simulink model "sim"  (R2016b)
settings: Solver=FixedStepDiscrete  StartTime=0  StopTime=Stoptime  FixedStep=0.1  RelTol=1e-3  EnableMultiTasking=on
values from neighbouring files (symbols this model uses):
  CYC_v = smooth(CYC_v,0.005 )    [main.m]
  ShiftDown = reshape(shift_down, [6,17])    [main.m]
  ShiftUp = reshape(shift_up, [5,17])    [main.m]
  VEH_M2 = 8700    [main.m]
undefined symbols (not defined in the file or in its folder): BrakeTorqueGain, CYC_gear, CYC_grade, CYC_t, DiscIntNeverNeededParam, DR_FF, DR_I, DR_P, Enable_Lag, Enable_Shift, ENG_Iei, Engine, Fr, g, ICE_maxT_T, ICE_maxT_w, Init, Powtrain_eff, sample_time, TC_Kfactor, TC_speedratio, TC_Torkratio, TRAN_gear, TRAN_ratio_diff, TRAN_ratio_gear, VEH_Cdl, VEH_M, VEH_Rw, WOT
libraries: simulink x2
settings Model: Creator=Dalaska  LastModifiedBy=daruiz
settings DataIOCC: LimitDataPoints=on  SaveFormat=Array
settings OptimizationCC: LifeSpan=inf
settings DebuggingCC: SFUnexpectedBacktrackingDiag=warning  SFNoUnconditionalDefaultTransitionDiag=warning  SFExecutionAtInitializationDiag=none
settings HardwareCC: ProdBitPerPointer=32  ProdBitPerSizeT=32  ProdBitPerPtrDiffT=32  ProdLargestAtomicFloat=None  ProdIntDivRoundTo=Undefined  ProdEndianess=Unspecified  ProdWordSize=32  ProdHWDeviceType=32-bit Generic
settings ModelReferenceCC: PropagateSignalLabelsOutOfModel=off
settings GRTTargetCC: TargetLangStandard=C89/C90 (ANSI)  GeneratePreprocessorConditionals=Disable all
settings ConfigComp: CovMetricSettings=dw  CovHtmlReporting=on  CovSaveCumulativeToWorkspaceVar=on  CovSaveSingleToWorkspaceVar=on  CovExternalEMLEnable=off

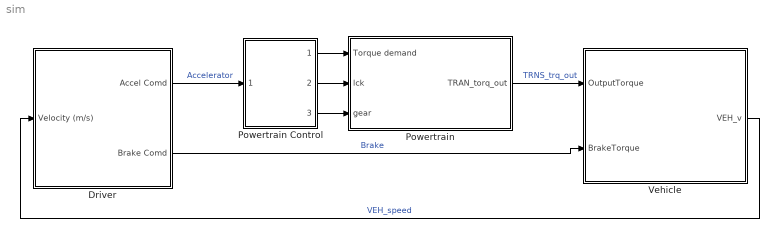
== system sim ==
  "Driver " : Subsystem
      mask Display: image(imread('Images\driver.jpg'))
  "Powertrain " : Subsystem
      mask Display: image(imread('Images\powertrain.jpg'))
  Powertrain Control : Subsystem
  Vehicle : Subsystem
      mask Display: image(imread('Images\truck.jpg'))
  wires:
  "Powertrain "/1(TRAN_torq_out) -> Vehicle/1(OutputTorque)  "TRNS_trq_out"
  "Driver "/1(Accel Comd) -> Powertrain Control/1(Throttle)  "Accelerator"
  Powertrain Control/1(ENG_torq) -> "Powertrain "/1(Torque demand)
  Powertrain Control/2(TC_lock) -> "Powertrain "/2(lck)
  Powertrain Control/3(TRAN_gear) -> "Powertrain "/3(gear)
  "Driver "/2(Brake Comd) -> Vehicle/2(BrakeTorque)  "Brake"
  Vehicle/1(VEH_v) -> "Driver "/1(Velocity (m/s))  "VEH_speed"

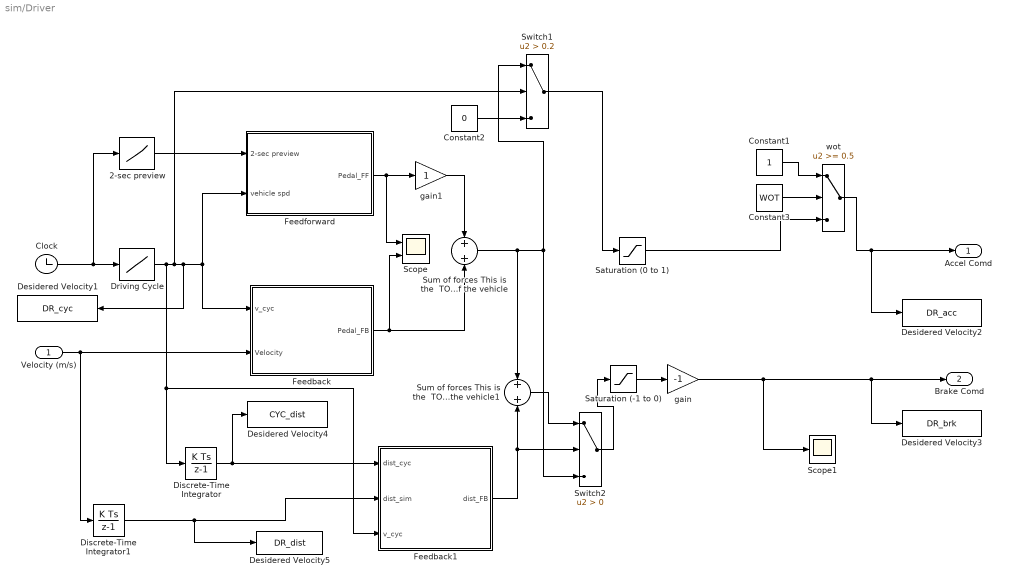
== system sim/Driver  ==
  Velocity (m/s) : Inport
  2-sec preview : Lookup  InputValues=CYC_t(1:length(CYC_t)-2)  Table=CYC_v(3:length(CYC_v))  SaturateOnIntegerOverflow=on
  Clock : Clock
  Constant1 : Constant
  Constant2 : Constant  Value=0
  Constant3 : Constant  Value=WOT
  Desidered Velocity1 : ToWorkspace  VariableName=DR_cyc  SaveFormat=Timeseries  SampleTime=-1
  Desidered Velocity2 : ToWorkspace  VariableName=DR_acc  SaveFormat=Timeseries  SampleTime=-1
  Desidered Velocity3 : ToWorkspace  VariableName=DR_brk  SaveFormat=Timeseries  SampleTime=-1
  Desidered Velocity4 : ToWorkspace  VariableName=CYC_dist  SaveFormat=Timeseries  SampleTime=-1
  Desidered Velocity5 : ToWorkspace  VariableName=DR_dist  SaveFormat=Timeseries  SampleTime=-1
  Discrete-Time Integrator : DiscreteIntegrator  InitialConditionSetting=State (most efficient)  SampleTime=sample_time  ICPrevOutput=DiscIntNeverNeededParam  ICPrevScaledInput=DiscIntNeverNeededParam
  Discrete-Time Integrator1 : DiscreteIntegrator  InitialConditionSetting=State (most efficient)  SampleTime=sample_time  ICPrevOutput=DiscIntNeverNeededParam  ICPrevScaledInput=DiscIntNeverNeededParam
  Driving Cycle : Lookup  InputValues=CYC_t  Table=CYC_v  SaturateOnIntegerOverflow=on
  Feedback : Subsystem
  Feedback1 : Subsystem
  Feedforward : Subsystem
  Saturation (-1 to 0) : Saturate  UpperLimit=0  LowerLimit=-1
  Saturation (0 to 1) : Saturate  UpperLimit=1  LowerLimit=0
  Scope : Scope  NumInputPorts=2
  Scope1 : Scope
  Sum of forces This is the  TOTAL force resisting forward motion of the vehicle : Sum  Tag=R12-1  SaturateOnIntegerOverflow=on  InputSameDT=on  OutDataTypeStr=Inherit: Same as first input
  Sum of forces This is the  TOTAL force resisting forward motion of the vehicle1 : Sum  Tag=R12-1  SaturateOnIntegerOverflow=on  InputSameDT=on  OutDataTypeStr=Inherit: Same as first input
  Switch1 : Switch  Criteria=u2 > Threshold  Threshold=0.2  SaturateOnIntegerOverflow=on  InputSameDT=on
  Switch2 : Switch  Criteria=u2 > Threshold  SaturateOnIntegerOverflow=on  InputSameDT=on
  gain : Gain  Gain=-1  SaturateOnIntegerOverflow=on  OutDataTypeStr=Inherit: Same as input  ParamDataTypeStr=Inherit: Same as input
  gain1 : Gain  SaturateOnIntegerOverflow=on  OutDataTypeStr=Inherit: Same as input  ParamDataTypeStr=Inherit: Same as input
  wot : Switch  Threshold=0.5
  Accel Comd : Outport  InitialOutput=0
  Brake Comd : Outport  Port=2  InitialOutput=0
  wires:
  Velocity (m/s)/1 -> Feedback/2(Velocity), Discrete-Time Integrator1/1
  Clock/1 -> 2-sec preview/1, Driving Cycle/1
  Driving Cycle/1 -> Switch1/2, Feedforward/2(vehicle spd), Feedback/1(v_cyc), Desidered Velocity1/1, Feedback1/3(v_cyc), Discrete-Time Integrator/1
  2-sec preview/1 -> Feedforward/1(2-sec preview)
  Feedforward/1(Pedal_FF) -> Scope/1, gain1/1
  Saturation (-1 to 0)/1 -> gain/1
  Feedback/1(Pedal_FB) -> Sum of forces This is the  TOTAL force resisting forward motion of the vehicle/2, Scope/2
  Discrete-Time Integrator/1 -> Desidered Velocity4/1, Feedback1/1(dist_cyc)
  Discrete-Time Integrator1/1 -> Feedback1/2(dist_sim), Desidered Velocity5/1
  Sum of forces This is the  TOTAL force resisting forward motion of the vehicle/1 -> Sum of forces This is the  TOTAL force resisting forward motion of the vehicle1/1, Switch1/1, Switch2/3
  gain/1 -> Scope1/1, Desidered Velocity3/1, Brake Comd/1
  gain1/1 -> Sum of forces This is the  TOTAL force resisting forward motion of the vehicle/1
  wot/1 -> Desidered Velocity2/1, Accel Comd/1
  Constant1/1 -> wot/1
  Constant3/1 -> wot/2
  Saturation (0 to 1)/1 -> wot/3
  Feedback1/1(dist_FB) -> Sum of forces This is the  TOTAL force resisting forward motion of the vehicle1/2, Switch2/2
  Sum of forces This is the  TOTAL force resisting forward motion of the vehicle1/1 -> Switch2/1
  Switch2/1 -> Saturation (-1 to 0)/1
  Switch1/1 -> Saturation (0 to 1)/1
  Constant2/1 -> Switch1/3

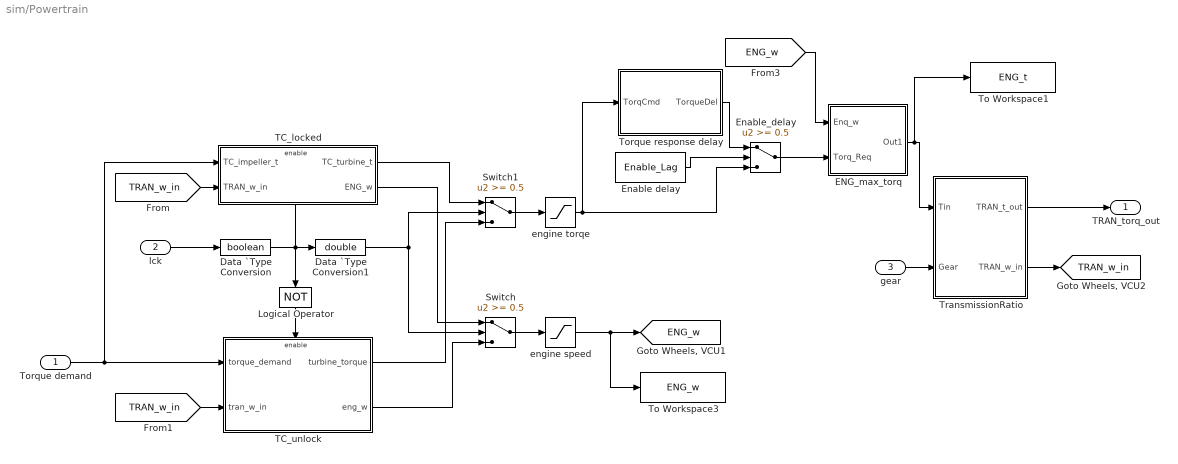
== system sim/Powertrain  ==
  Torque demand : Inport
  lck : Inport  Port=2
  gear : Inport  Port=3
  Data `Type Conversion : DataTypeConversion  OutDataTypeStr=boolean
  Data `Type Conversion1 : DataTypeConversion  OutDataTypeStr=double
  ENG_max_torq : Subsystem
  Enable delay : Constant  Value=Enable_Lag
  Enable_delay : Switch  Threshold=0.5
  Logical Operator : Logic  Operator=NOT  AllPortsSameDT=off  OutDataTypeStr=boolean
  Switch : Switch  Threshold=0.5
  Switch1 : Switch  Threshold=0.5
  TC_locked : Subsystem
  TC_unlock : Subsystem
  To Workspace1 : ToWorkspace  VariableName=ENG_t  SaveFormat=Timeseries  SampleTime=-1
  To Workspace3 : ToWorkspace  VariableName=ENG_w  SaveFormat=Timeseries  SampleTime=-1
  Torque response delay : Subsystem
  TransmissionRatio : Subsystem
  engine speed : Saturate  UpperLimit=2800  LowerLimit=700
  engine torqe : Saturate  UpperLimit=610  LowerLimit=0
  TRAN_torq_out : Outport
  tag scope: ENG_w=global, TRAN_w_in=global
  wires:
  gear/1 -> TransmissionRatio/2(Gear)
  TransmissionRatio/1("TRAN_t_out ") -> TRAN_torq_out/1
  lck/1 -> Data `Type Conversion/1
  TC_locked/2(ENG_w) -> Switch/1
  Data `Type Conversion/1 -> Logical Operator/1, Data `Type Conversion1/1, TC_locked/Enable
  Data `Type Conversion1/1 -> Switch/2, Switch1/2
  Logical Operator/1 -> TC_unlock/Enable
  TC_locked/1("TC_turbine_t ") -> Switch1/1
  TC_unlock/1(turbine_torque) -> Switch1/3
  TC_unlock/2(eng_w) -> Switch/3
  Switch/1 -> engine speed/1
  engine speed/1 -> [ENG_w], To Workspace3/1
  Torque demand/1 -> TC_locked/1(TC_impeller_t), TC_unlock/1(torque_demand)
  TransmissionRatio/2(TRAN_w_in) -> [TRAN_w_in]
  [TRAN_w_in] -> TC_locked/2(TRAN_w_in)
  [TRAN_w_in] -> TC_unlock/2(tran_w_in)
  ENG_max_torq/1(Out1) -> TransmissionRatio/1(Tin), To Workspace1/1
  Torque response delay/1(TorqueDel) -> Enable_delay/1
  Enable delay/1 -> Enable_delay/2
  [ENG_w] -> ENG_max_torq/1(Enq_w)
  Switch1/1 -> engine torqe/1
  Enable_delay/1 -> ENG_max_torq/2(Torq_Req)
  engine torqe/1 -> Enable_delay/3, Torque response delay/1(TorqCmd)

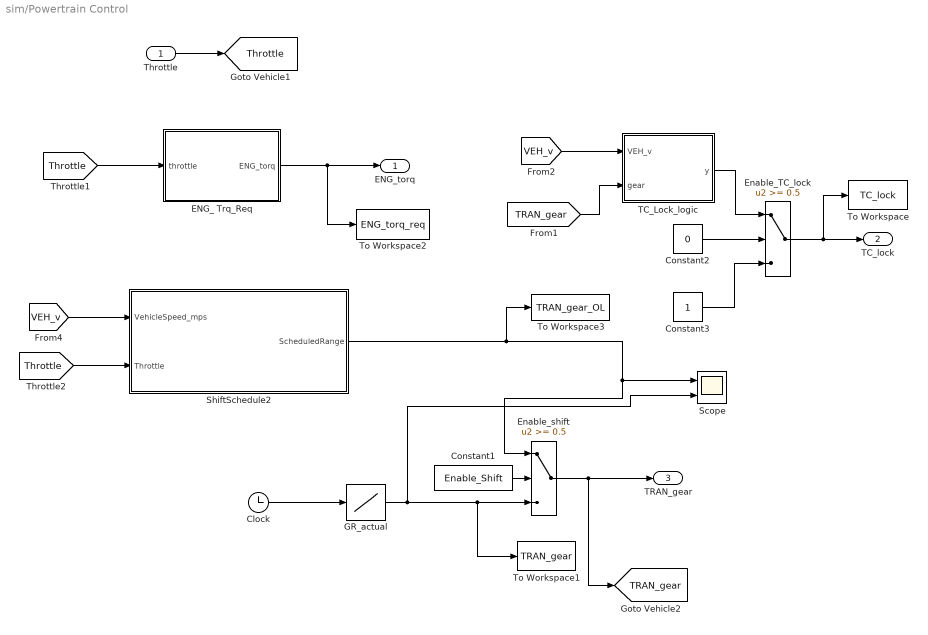
== system sim/Powertrain Control ==
  Throttle : Inport
  Clock : Clock
  Constant1 : Constant  Value=Enable_Shift
  Constant2 : Constant  Value=0
  Constant3 : Constant
  ENG_ Trq_Req : Subsystem
  Enable_TC_lock : Switch  Threshold=0.5
  Enable_shift : Switch  Threshold=0.5
  GR_actual : Lookup  InputValues=CYC_t  Table=CYC_gear  LookUpMeth=Use Input Nearest  SaturateOnIntegerOverflow=on
  Scope : Scope  NumInputPorts=2
  ShiftSchedule2 : Subsystem  TreatAsAtomicUnit=on
  TC_Lock_logic : MATLAB Function  TreatAsAtomicUnit=on
  To Workspace : ToWorkspace  VariableName=TC_lock  SaveFormat=Timeseries  SampleTime=-1
  To Workspace1 : ToWorkspace  VariableName=TRAN_gear  SaveFormat=Timeseries  SampleTime=-1
  To Workspace2 : ToWorkspace  VariableName=ENG_torq_req  SaveFormat=Timeseries  SampleTime=-1
  To Workspace3 : ToWorkspace  VariableName=TRAN_gear_OL  SaveFormat=Timeseries  SampleTime=-1
  ENG_torq : Outport
  TC_lock : Outport  Port=2
  TRAN_gear : Outport  Port=3
  tag scope: TRAN_gear=global, Throttle=global
  wires:
  Throttle/1 -> [Throttle]
  ENG_ Trq_Req/1(ENG_torq) -> ENG_torq/1, To Workspace2/1
  [VEH_v] -> TC_Lock_logic/1(VEH_v)
  Enable_shift/1 -> [TRAN_gear], TRAN_gear/1
  Clock/1 -> GR_actual/1
  GR_actual/1 -> Enable_shift/3, To Workspace1/1, Scope/2
  ShiftSchedule2/1(ScheduledRange) -> To Workspace3/1, Scope/1, Enable_shift/1
  Constant1/1 -> Enable_shift/2
  [TRAN_gear] -> TC_Lock_logic/2(gear)
  Constant3/1 -> Enable_TC_lock/3
  Enable_TC_lock/1 -> TC_lock/1, To Workspace/1
  Constant2/1 -> Enable_TC_lock/2
  TC_Lock_logic/1(y) -> Enable_TC_lock/1
  [Throttle] -> ENG_ Trq_Req/1(throttle)
  [VEH_v] -> ShiftSchedule2/1(VehicleSpeed_mps)
  [Throttle] -> ShiftSchedule2/2(Throttle)

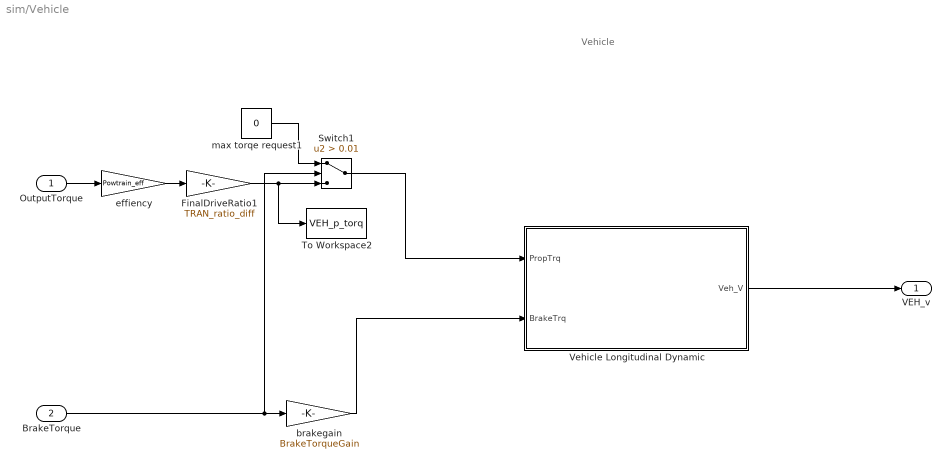
== system sim/Vehicle ==
  note: Vehicle
  OutputTorque : Inport
  BrakeTorque : Inport  Port=2
  FinalDriveRatio1 : Gain  Gain=TRAN_ratio_diff  SaturateOnIntegerOverflow=on  OutDataTypeStr=Inherit: Same as input  ParamDataTypeStr=Inherit: Same as input
  Switch1 : Switch  Criteria=u2 > Threshold  Threshold=0.01  ZeroCross=off
  To Workspace2 : ToWorkspace  VariableName=VEH_p_torq  SaveFormat=Timeseries  SampleTime=-1
  Vehicle Longitudinal Dynamic : Subsystem
  brakegain : Gain  Gain=BrakeTorqueGain  SaturateOnIntegerOverflow=on  OutDataTypeStr=Inherit: Same as input  ParamDataTypeStr=Inherit: Same as input
  effiency : Gain  Gain=Powtrain_eff  SaturateOnIntegerOverflow=on  OutDataTypeStr=Inherit: Same as input  ParamDataTypeStr=Inherit: Same as input
  max torqe request1 : Constant  Value=0  SampleTime=0
  VEH_v : Outport
  wires:
  OutputTorque/1 -> effiency/1
  BrakeTorque/1 -> Switch1/2, brakegain/1
  FinalDriveRatio1/1 -> To Workspace2/1, Switch1/3
  max torqe request1/1 -> Switch1/1
  effiency/1 -> FinalDriveRatio1/1
  Switch1/1 -> Vehicle Longitudinal Dynamic/1(PropTrq)
  brakegain/1 -> Vehicle Longitudinal Dynamic/2(BrakeTrq)
  Vehicle Longitudinal Dynamic/1(Veh_V) -> VEH_v/1

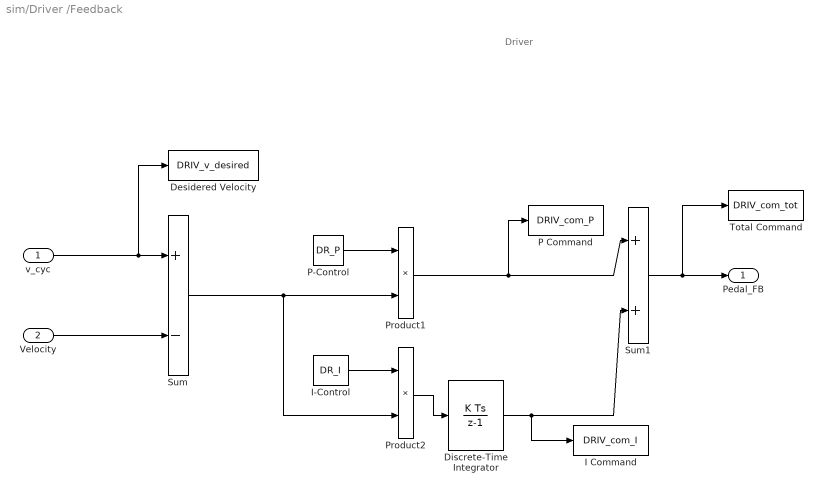
== system sim/Driver /Feedback ==
  note: Driver
  v_cyc : Inport
  Velocity : Inport  Port=2
  Desidered Velocity : ToWorkspace  VariableName=DRIV_v_desired  SampleTime=-1
  Discrete-Time Integrator : DiscreteIntegrator  InitialConditionSetting=State (most efficient)  SampleTime=sample_time  ICPrevOutput=DiscIntNeverNeededParam  ICPrevScaledInput=DiscIntNeverNeededParam
  I Command : ToWorkspace  VariableName=DRIV_com_I  SampleTime=-1
  I-Control : Constant  Value=DR_I
  P Command : ToWorkspace  VariableName=DRIV_com_P  SampleTime=-1
  P-Control : Constant  Value=DR_P
  Product1 : Product  RndMeth=Zero
  Product2 : Product  RndMeth=Zero
  Sum : Sum  Inputs=+-  SaturateOnIntegerOverflow=on  InputSameDT=on  OutDataTypeStr=Inherit: Same as first input
  Sum1 : Sum  SaturateOnIntegerOverflow=on  InputSameDT=on  OutDataTypeStr=Inherit: Same as first input
  Total Command : ToWorkspace  VariableName=DRIV_com_tot  SampleTime=-1
  Pedal_FB : Outport
  wires:
  Sum1/1 -> Total Command/1, Pedal_FB/1
  Sum/1 -> Product1/2, Product2/2
  Product1/1 -> Sum1/1, P Command/1
  Product2/1 -> Discrete-Time Integrator/1
  Discrete-Time Integrator/1 -> I Command/1, Sum1/2
  P-Control/1 -> Product1/1
  v_cyc/1 -> Sum/1, Desidered Velocity/1
  I-Control/1 -> Product2/1
  Velocity/1 -> Sum/2

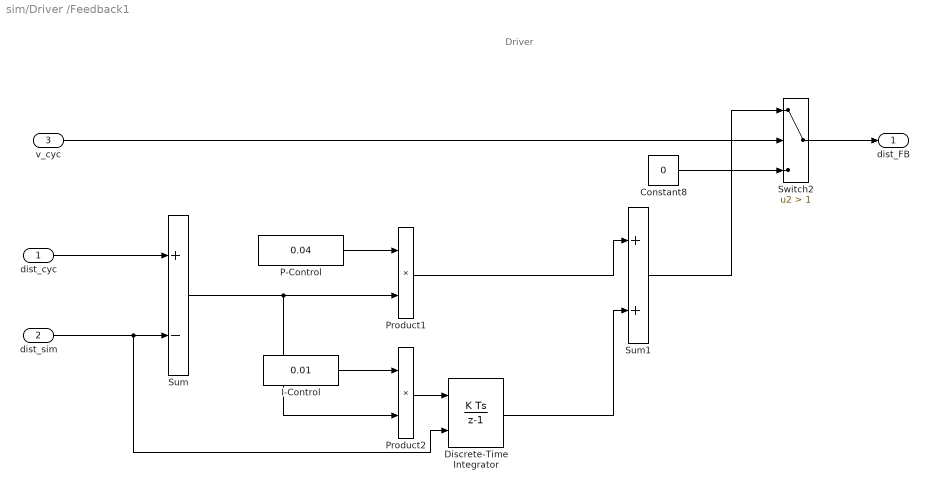
== system sim/Driver /Feedback1 ==
  note: Driver
  dist_cyc : Inport
  dist_sim : Inport  Port=2
  v_cyc : Inport  Port=3
  Constant8 : Constant  Value=0
  Discrete-Time Integrator : DiscreteIntegrator  ExternalReset=level  InitialConditionSetting=State (most efficient)  SampleTime=sample_time  ICPrevOutput=DiscIntNeverNeededParam  ICPrevScaledInput=DiscIntNeverNeededParam
  I-Control : Constant  Value=0.01
  P-Control : Constant  Value=0.04
  Product1 : Product  RndMeth=Zero
  Product2 : Product  RndMeth=Zero
  Sum : Sum  Inputs=+-  SaturateOnIntegerOverflow=on  InputSameDT=on  OutDataTypeStr=Inherit: Same as first input
  Sum1 : Sum  SaturateOnIntegerOverflow=on  InputSameDT=on  OutDataTypeStr=Inherit: Same as first input
  Switch2 : Switch  Criteria=u2 > Threshold  Threshold=1  SaturateOnIntegerOverflow=on  InputSameDT=on
  dist_FB : Outport
  wires:
  dist_sim/1 -> Discrete-Time Integrator/2, Sum/2
  Sum/1 -> Product1/2, Product2/2
  Product1/1 -> Sum1/1
  Product2/1 -> Discrete-Time Integrator/1
  Discrete-Time Integrator/1 -> Sum1/2
  P-Control/1 -> Product1/1
  dist_cyc/1 -> Sum/1
  I-Control/1 -> Product2/1
  v_cyc/1 -> Switch2/2
  Switch2/1 -> dist_FB/1
  Constant8/1 -> Switch2/3
  Sum1/1 -> Switch2/1

== system sim/Driver /Feedforward ==
  2-sec preview : Inport
  vehicle spd : Inport  Port=2
  Preview Gain : Gain  Gain=DR_FF  SaturateOnIntegerOverflow=on  OutDataTypeStr=Inherit: Same as input  ParamDataTypeStr=Inherit: Same as input
  Sum1 : Sum  Inputs=|+-  SaturateOnIntegerOverflow=on  InputSameDT=on  OutDataTypeStr=Inherit: Same as first input
  Pedal_FF : Outport
  wires:
  2-sec preview/1 -> Sum1/1
  Sum1/1 -> Preview Gain/1
  Preview Gain/1 -> Pedal_FF/1
  vehicle spd/1 -> Sum1/2

== system sim/Powertrain /ENG_max_torq ==
  Enq_w : Inport
  Torq_Req : Inport  Port=2
  Constant3 : Constant  Value=0
  ICE Max Torque Curve : Lookup  InputValues=ICE_maxT_w  Table=ICE_maxT_T  SaturateOnIntegerOverflow=on
  Saturation Dynamic : simulink/Discontinuities/Saturation Dynamic  OutMin=[]  OutMax=[]  OutDataTypeStr=Inherit: Same as second input  OutDataType=sfix(16)  OutScaling=2^-10  DoSatur=off
  rpm 2 rad/sec : Gain  Gain=pi*2/60
  Out1 : Outport
  wires:
  Saturation Dynamic/1 -> Out1/1
  rpm 2 rad/sec/1 -> ICE Max Torque Curve/1
  Constant3/1 -> Saturation Dynamic/3
  ICE Max Torque Curve/1 -> Saturation Dynamic/1
  Torq_Req/1 -> Saturation Dynamic/2
  Enq_w/1 -> rpm 2 rad/sec/1

== system sim/Powertrain /TC_locked ==
  TC_impeller_t : Inport
  TRAN_w_in : Inport  Port=2
  Enable : EnablePort  StatesWhenEnabling=reset  PropagateVarSize=During execution
  "TC_turbine_t " : Outport
  ENG_w : Outport  Port=2
  wires:
  TC_impeller_t/1 -> "TC_turbine_t "/1
  TRAN_w_in/1 -> ENG_w/1

== system sim/Powertrain /TC_unlock ==
  torque_demand : Inport
  tran_w_in : Inport  Port=2
  Enable : EnablePort  StatesWhenEnabling=reset  PropagateVarSize=During execution
  TC : Subsystem
  engine : Subsystem
  turbine_torque : Outport
  eng_w : Outport  Port=2
  wires:
  torque_demand/1 -> engine/2(Torque_Demand)
  TC/1("TC_impeller_t ") -> engine/1(Torque_Break)
  engine/1(ENG_w) -> eng_w/1, TC/1(TC_impeller_w)
  TC/2("TC_turbine_t ") -> turbine_torque/1  "TurbineTorque"
  tran_w_in/1 -> TC/2(TC_trub_w)

== system sim/Powertrain /Torque response delay ==
  TorqCmd : Inport  OutDataTypeStr=double  PortDimensions=1
  1-D Lookup Table : Lookup_n-D  NumberOfTableDimensions=1  BreakpointsForDimension1=[600 1200]  Table=[.8333 .8333]  ExtrapMethod=Clip  UseLastTableValue=on  RndMeth=Simplest  InputSameDT=on
  1-D Lookup Table1 : Lookup_n-D  NumberOfTableDimensions=1  BreakpointsForDimension1=[-.1 500]  Table=[10 .8333]  ExtrapMethod=Clip  UseLastTableValue=on  RndMeth=Simplest  InputSameDT=on
  Constant : Constant  Value=10  OutDataTypeStr=double
  Discrete Transfer Fcn (need to update coefficients) : DiscreteTransferFcn  Numerator=Engine.TorqResponseFltrNum  Denominator=Engine.TorqResponseFltrDen  SampleTime=sample_time
  Relational Operator : RelationalOperator  Operator=<=  OutDataTypeStr=boolean  RndMeth=Nearest
  Select Max : MinMax  Function=max  Inputs=2
  Switch : Switch  Criteria=u2 ~= 0
  Variable Rate Discrete Lag Filter : Subsystem
  TorqueDel : Outport
  wires:
  Variable Rate Discrete Lag Filter/1(Output) -> TorqueDel/1, 1-D Lookup Table1/1, Discrete Transfer Fcn (need to update coefficients)/1
  TorqCmd/1 -> Relational Operator/1, Variable Rate Discrete Lag Filter/1(Input)
  Discrete Transfer Fcn (need to update coefficients)/1 -> 1-D Lookup Table/1, Relational Operator/2
  Switch/1 -> Variable Rate Discrete Lag Filter/2(wn)
  Relational Operator/1 -> Switch/2
  Constant/1 -> Switch/1
  1-D Lookup Table/1 -> Select Max/2
  Select Max/1 -> Switch/3
  1-D Lookup Table1/1 -> Select Max/1

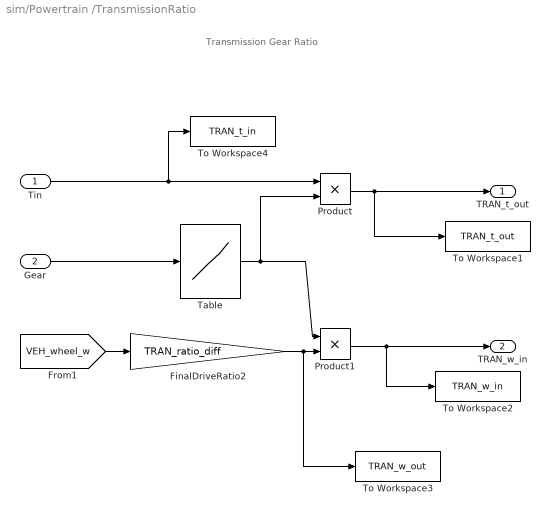
== system sim/Powertrain /TransmissionRatio ==
  note: Transmission Gear Ratio
  Tin : Inport
  Gear : Inport  Port=2
  FinalDriveRatio2 : Gain  Gain=TRAN_ratio_diff  SaturateOnIntegerOverflow=on  OutDataTypeStr=Inherit: Same as input  ParamDataTypeStr=Inherit: Same as input
  Product : Product  SaturateOnIntegerOverflow=on  InputSameDT=on  OutDataTypeStr=Inherit: Same as first input
  Product1 : Product  SaturateOnIntegerOverflow=on  InputSameDT=on  OutDataTypeStr=Inherit: Same as first input
  Table : Lookup_n-D  NumberOfTableDimensions=1  BreakpointsForDimension1=TRAN_gear  Table=TRAN_ratio_gear  OutDataTypeStr=double  SaturateOnIntegerOverflow=on  InputSameDT=on  LockScale=on
  To Workspace1 : ToWorkspace  VariableName=TRAN_t_out  SaveFormat=Timeseries  SampleTime=-1
  To Workspace2 : ToWorkspace  VariableName=TRAN_w_in  SaveFormat=Timeseries  SampleTime=-1
  To Workspace3 : ToWorkspace  VariableName=TRAN_w_out  SaveFormat=Timeseries  SampleTime=-1
  To Workspace4 : ToWorkspace  VariableName=TRAN_t_in  SaveFormat=Timeseries  SampleTime=-1
  "TRAN_t_out " : Outport
  TRAN_w_in : Outport  Port=2
  wires:
  Table/1 -> Product1/1, Product/2
  Tin/1 -> To Workspace4/1, Product/1
  Gear/1 -> Table/1
  [VEH_wheel_w] -> FinalDriveRatio2/1
  Product/1 -> To Workspace1/1, "TRAN_t_out "/1
  FinalDriveRatio2/1 -> To Workspace3/1, Product1/2
  Product1/1 -> TRAN_w_in/1, To Workspace2/1

== system sim/Powertrain Control/ENG_ Trq_Req ==
  throttle : Inport
  ENG_max_torq : Subsystem
  Max_torqe_request : Constant  Value=620
  Memory : Memory
  Product3 : Product  RndMeth=Zero
  ENG_torq : Outport
  wires:
  [ENG_w] -> Memory/1
  Memory/1 -> ENG_max_torq/1(Enq_w)
  throttle/1 -> Product3/1
  ENG_max_torq/1(Out1) -> ENG_torq/1
  Max_torqe_request/1 -> Product3/2
  Product3/1 -> ENG_max_torq/2(Torq_Req)

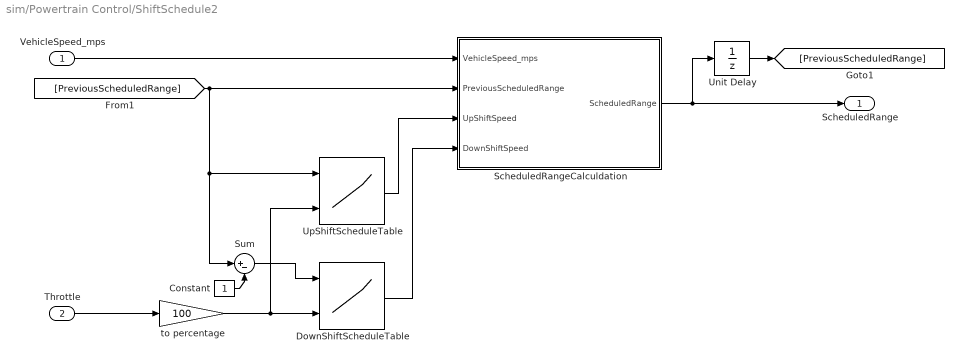
== system sim/Powertrain Control/ShiftSchedule2 ==
  VehicleSpeed_mps : Inport  OutDataTypeStr=double  PortDimensions=1
  Throttle : Inport  Port=2  OutDataTypeStr=double  PortDimensions=1
  Constant : Constant
  DownShiftScheduleTable : Lookup_n-D  BreakpointsForDimension1=[0:1:5]  BreakpointsForDimension2=[0:6.25:100]  BeginIndexSearchUsingPreviousIndexResult=on  Table=ShiftDown  ExtrapMethod=Clip  UseLastTableValue=on  RndMeth=Simplest  InputSameDT=on
  ScheduledRangeCalculdation : Subsystem  TreatAsAtomicUnit=on
  Sum : Sum  Inputs=|+-
  Unit Delay : UnitDelay  InitialCondition=1  SampleTime=-1
  UpShiftScheduleTable : Lookup_n-D  BreakpointsForDimension1=[1:1:5]  BreakpointsForDimension2=[0:6.25:100]  BeginIndexSearchUsingPreviousIndexResult=on  Table=ShiftUp  ExtrapMethod=Clip  UseLastTableValue=on  RndMeth=Simplest  InputSameDT=on
  to percentage : Gain  Gain=100  SaturateOnIntegerOverflow=on  OutDataTypeStr=Inherit: Same as input  ParamDataTypeStr=Inherit: Same as input
  ScheduledRange : Outport  OutDataTypeStr=double  PortDimensions=1
  wires:
  ScheduledRangeCalculdation/1(ScheduledRange) -> Unit Delay/1, ScheduledRange/1
  VehicleSpeed_mps/1 -> ScheduledRangeCalculdation/1(VehicleSpeed_mps)
  DownShiftScheduleTable/1 -> ScheduledRangeCalculdation/4(DownShiftSpeed)
  UpShiftScheduleTable/1 -> ScheduledRangeCalculdation/3(UpShiftSpeed)
  Throttle/1 -> to percentage/1
  to percentage/1 -> UpShiftScheduleTable/2, DownShiftScheduleTable/2
  Unit Delay/1 -> [PreviousScheduledRange]
  [PreviousScheduledRange] -> ScheduledRangeCalculdation/2(PreviousScheduledRange), Sum/1, UpShiftScheduleTable/1
  Sum/1 -> DownShiftScheduleTable/1
  Constant/1 -> Sum/2

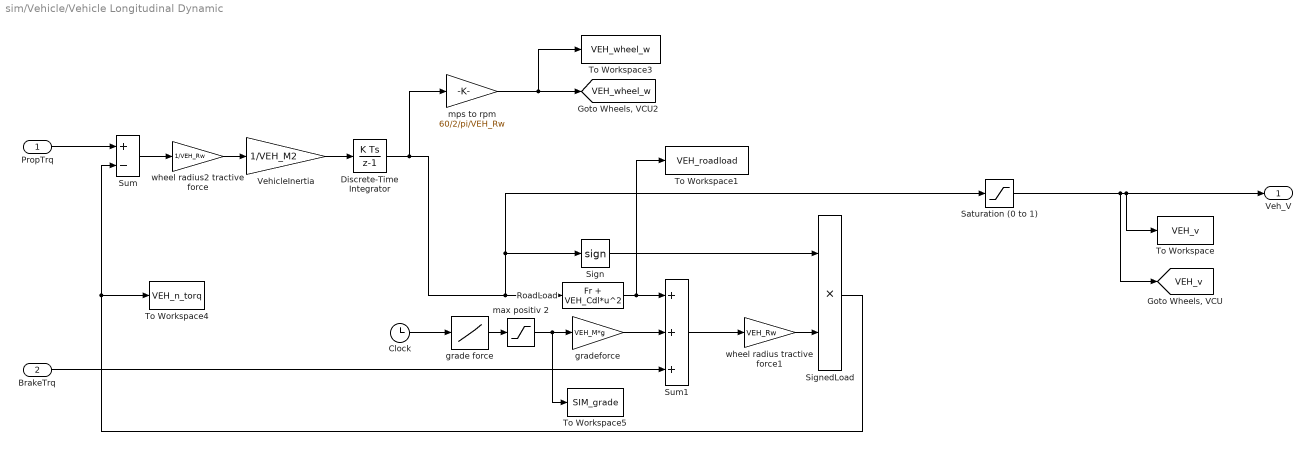
== system sim/Vehicle/Vehicle Longitudinal Dynamic ==
  PropTrq : Inport
  BrakeTrq : Inport  Port=2
  Clock : Clock
  Discrete-Time Integrator : DiscreteIntegrator  InitialConditionSetting=State (most efficient)  SampleTime=sample_time  ICPrevOutput=DiscIntNeverNeededParam  ICPrevScaledInput=DiscIntNeverNeededParam
  RoadLoad : Fcn  Expr=Fr + VEH_Cdl*u^2
  Saturation (0 to 1) : Saturate  UpperLimit=100  LowerLimit=0
  Sign : Signum
  SignedLoad : Product  SaturateOnIntegerOverflow=on  InputSameDT=on  OutDataTypeStr=Inherit: Same as first input
  Sum : Sum  Inputs=+-  SaturateOnIntegerOverflow=on  InputSameDT=on  OutDataTypeStr=Inherit: Same as first input
  Sum1 : Sum  Inputs=+++  SaturateOnIntegerOverflow=on  InputSameDT=on  OutDataTypeStr=Inherit: Same as first input
  To Workspace : ToWorkspace  VariableName=VEH_v  SaveFormat=Timeseries  SampleTime=-1
  To Workspace1 : ToWorkspace  VariableName=VEH_roadload  SaveFormat=Timeseries  SampleTime=-1
  To Workspace3 : ToWorkspace  VariableName=VEH_wheel_w  SaveFormat=Timeseries  SampleTime=-1
  To Workspace4 : ToWorkspace  VariableName=VEH_n_torq  SaveFormat=Timeseries  SampleTime=-1
  To Workspace5 : ToWorkspace  VariableName=SIM_grade  SaveFormat=Timeseries  SampleTime=-1
  VehicleInertia : Gain  Gain=1/VEH_M2  SaturateOnIntegerOverflow=on  OutDataTypeStr=Inherit: Same as input  ParamDataTypeStr=Inherit: Same as input
  grade force : Lookup  InputValues=CYC_t  Table=CYC_grade  SaturateOnIntegerOverflow=on
  gradeforce : Gain  Gain=VEH_M*g  SaturateOnIntegerOverflow=on  OutDataTypeStr=Inherit: Same as input  ParamDataTypeStr=Inherit: Same as input
  max positiv 2 : Saturate  UpperLimit=0.01  LowerLimit=-0.05
  mps to rpm : Gain  Gain=60/2/pi/VEH_Rw  SaturateOnIntegerOverflow=on  OutDataTypeStr=Inherit: Same as input  ParamDataTypeStr=Inherit: Same as input
  wheel radius tractive force1 : Gain  Gain=VEH_Rw  SaturateOnIntegerOverflow=on  OutDataTypeStr=Inherit: Same as input  ParamDataTypeStr=Inherit: Same as input
  wheel radius2 tractive force : Gain  Gain=1/VEH_Rw  SaturateOnIntegerOverflow=on  OutDataTypeStr=Inherit: Same as input  ParamDataTypeStr=Inherit: Same as input
  Veh_V : Outport
  tag scope: VEH_v=global, VEH_wheel_w=global
  wires:
  RoadLoad/1 -> Sum1/1, To Workspace1/1
  wheel radius2 tractive force/1 -> VehicleInertia/1
  VehicleInertia/1 -> Discrete-Time Integrator/1
  mps to rpm/1 -> [VEH_wheel_w], To Workspace3/1
  Sum1/1 -> wheel radius tractive force1/1
  Sign/1 -> SignedLoad/1
  Sum/1 -> wheel radius2 tractive force/1
  SignedLoad/1 -> Sum/2, To Workspace4/1
  BrakeTrq/1 -> Sum1/3
  PropTrq/1 -> Sum/1
  Clock/1 -> grade force/1
  Discrete-Time Integrator/1 -> Sign/1, Saturation (0 to 1)/1, RoadLoad/1, mps to rpm/1
  grade force/1 -> max positiv 2/1
  wheel radius tractive force1/1 -> SignedLoad/2
  max positiv 2/1 -> gradeforce/1, To Workspace5/1
  gradeforce/1 -> Sum1/2
  Saturation (0 to 1)/1 -> Veh_V/1, To Workspace/1, [VEH_v]

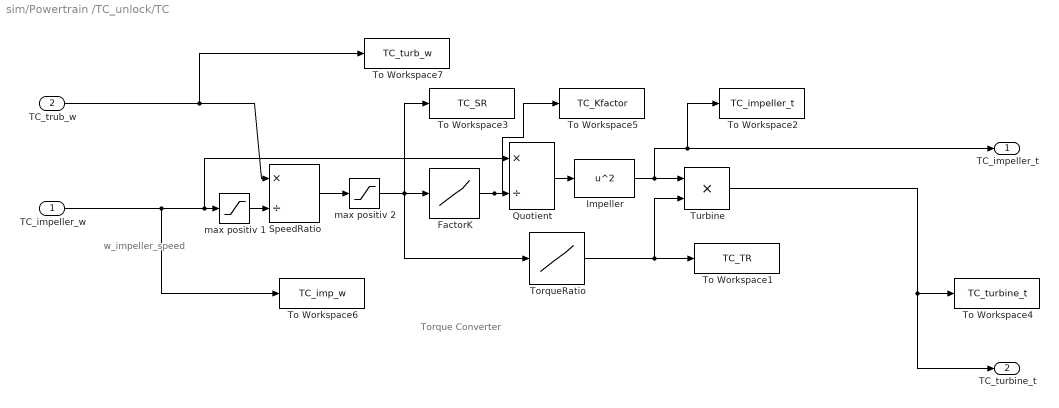
== system sim/Powertrain /TC_unlock/TC ==
  note: w_impeller_speed
  note: Torque Converter
  TC_impeller_w : Inport
  TC_trub_w : Inport  Port=2
  FactorK : Lookup_n-D  NumberOfTableDimensions=1  BreakpointsForDimension1=TC_speedratio  Table=TC_Kfactor  SaturateOnIntegerOverflow=on  InputSameDT=on
  Impeller : Fcn  Expr=u^2
  Quotient : Product  Inputs=*/  SaturateOnIntegerOverflow=on  InputSameDT=on  OutDataTypeStr=Inherit: Same as first input
  SpeedRatio : Product  Inputs=*/  SaturateOnIntegerOverflow=on  InputSameDT=on  OutDataTypeStr=Inherit: Same as first input
  To Workspace1 : ToWorkspace  VariableName=TC_TR  SaveFormat=Timeseries  SampleTime=-1
  To Workspace2 : ToWorkspace  VariableName=TC_impeller_t  SaveFormat=Timeseries  SampleTime=-1
  To Workspace3 : ToWorkspace  VariableName=TC_SR  SaveFormat=Timeseries  SampleTime=-1
  To Workspace4 : ToWorkspace  VariableName=TC_turbine_t  SaveFormat=Timeseries  SampleTime=-1
  To Workspace5 : ToWorkspace  VariableName=TC_Kfactor  SaveFormat=Timeseries  SampleTime=-1
  To Workspace6 : ToWorkspace  VariableName=TC_imp_w  SaveFormat=Timeseries  SampleTime=-1
  To Workspace7 : ToWorkspace  VariableName=TC_turb_w  SaveFormat=Timeseries  SampleTime=-1
  TorqueRatio : Lookup_n-D  NumberOfTableDimensions=1  BreakpointsForDimension1=TC_speedratio  Table=TC_Torkratio  SaturateOnIntegerOverflow=on  InputSameDT=on
  Turbine : Product  SaturateOnIntegerOverflow=on  InputSameDT=on  OutDataTypeStr=Inherit: Same as first input
  max positiv 1 : Saturate  UpperLimit=1000000  LowerLimit=0.1
  max positiv 2 : Saturate  UpperLimit=1  LowerLimit=0
  "TC_impeller_t " : Outport
  "TC_turbine_t " : Outport  Port=2
  wires:
  TorqueRatio/1 -> Turbine/2, To Workspace1/1
  Quotient/1 -> Impeller/1
  Impeller/1 -> "TC_impeller_t "/1, To Workspace2/1, Turbine/1
  SpeedRatio/1 -> max positiv 2/1
  FactorK/1 -> To Workspace5/1, Quotient/2
  Turbine/1 -> "TC_turbine_t "/1, To Workspace4/1
  max positiv 1/1 -> SpeedRatio/2
  TC_impeller_w/1 -> To Workspace6/1, Quotient/1, max positiv 1/1
  TC_trub_w/1 -> To Workspace7/1, SpeedRatio/1
  max positiv 2/1 -> FactorK/1, To Workspace3/1, TorqueRatio/1

== system sim/Powertrain /TC_unlock/engine ==
  note: Engine
  Torque_Break : Inport
  Torque_Demand : Inport  Port=2
  Discrete-Time Integrator : DiscreteIntegrator  InitialCondition=700  InitialConditionSetting=State (most efficient)  SampleTime=sample_time  ICPrevOutput=DiscIntNeverNeededParam  ICPrevScaledInput=DiscIntNeverNeededParam
  EnginePlusImpellerInertia : Gain  Gain=1/ENG_Iei  SaturateOnIntegerOverflow=on  OutDataTypeStr=Inherit: Same as input  ParamDataTypeStr=Inherit: Same as input
  Scope : Scope
  Sum : Sum  Inputs=-+  SaturateOnIntegerOverflow=on  InputSameDT=on  OutDataTypeStr=Inherit: Same as first input
  To Workspace1 : ToWorkspace  VariableName=ENG_brk_torq  SaveFormat=Timeseries  SampleTime=-1
  To Workspace2 : ToWorkspace  VariableName=ENG_dmnd_torq  SaveFormat=Timeseries  SampleTime=-1
  max positiv 1 : Saturate  UpperLimit=2600  LowerLimit=0.1
  ENG_w : Outport
  wires:
  Torque_Break/1 -> To Workspace1/1, Sum/1
  EnginePlusImpellerInertia/1 -> Discrete-Time Integrator/1
  Sum/1 -> EnginePlusImpellerInertia/1
  Torque_Demand/1 -> To Workspace2/1, Sum/2
  Discrete-Time Integrator/1 -> Scope/1, max positiv 1/1
  max positiv 1/1 -> ENG_w/1

== system sim/Powertrain /Torque response delay/Variable Rate Discrete Lag Filter ==
  Input : Inport
  wn : Inport  Port=2
  Discrete-Time Integrator : DiscreteIntegrator  InitialCondition=Init.EngineTorque  SampleTime=sample_time  ICPrevOutput=DiscIntNeverNeededParam  ICPrevScaledInput=DiscIntNeverNeededParam
  Sum3 : Sum  Inputs=-+|
  wn1 : Product  RndMeth=Zero
  Output : Outport
  wires:
  Input/1 -> Sum3/2
  wn/1 -> wn1/2
  Discrete-Time Integrator/1 -> Output/1, Sum3/1
  wn1/1 -> Discrete-Time Integrator/1
  Sum3/1 -> wn1/1

== system sim/Powertrain Control/ENG_ Trq_Req/ENG_max_torq ==
  Enq_w : Inport
  Torq_Req : Inport  Port=2
  Constant3 : Constant  Value=0
  ICE Max Torque Curve : Lookup  InputValues=ICE_maxT_w  Table=ICE_maxT_T  SaturateOnIntegerOverflow=on
  Saturation Dynamic : simulink/Discontinuities/Saturation Dynamic  OutMin=[]  OutMax=[]  OutDataTypeStr=Inherit: Same as second input  OutDataType=sfix(16)  OutScaling=2^-10  DoSatur=off
  To Workspace2 : ToWorkspace  VariableName=ENG_Max_t  SaveFormat=Timeseries  SampleTime=-1
  rpm 2 rad/sec : Gain  Gain=pi*2/60
  Out1 : Outport
  wires:
  Saturation Dynamic/1 -> Out1/1
  rpm 2 rad/sec/1 -> ICE Max Torque Curve/1
  Constant3/1 -> Saturation Dynamic/3
  ICE Max Torque Curve/1 -> To Workspace2/1, Saturation Dynamic/1
  Torq_Req/1 -> Saturation Dynamic/2
  Enq_w/1 -> rpm 2 rad/sec/1

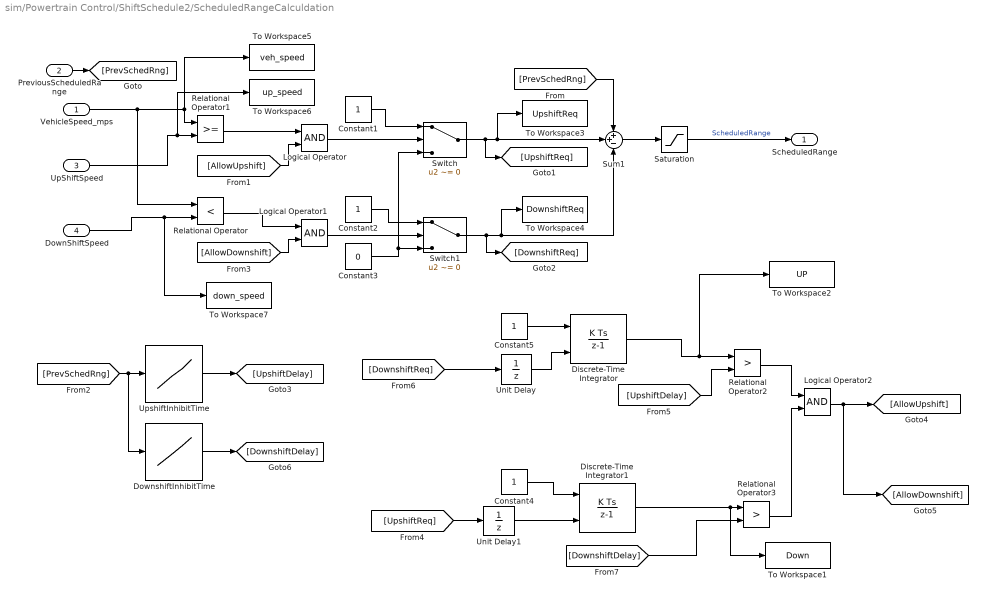
== system sim/Powertrain Control/ShiftSchedule2/ScheduledRangeCalculdation ==
  VehicleSpeed_mps : Inport
  PreviousScheduledRange : Inport  Port=2
  UpShiftSpeed : Inport  Port=3
  DownShiftSpeed : Inport  Port=4
  Constant{1..2,4..5} (4 alike) : Constant
  Constant3 : Constant  Value=0
  Discrete-Time Integrator : DiscreteIntegrator  ExternalReset=rising  SampleTime=0.1  LimitOutput=on  LowerSaturationLimit=0  ICPrevOutput=DiscIntNeverNeededParam  ICPrevScaledInput=DiscIntNeverNeededParam
  Discrete-Time Integrator1 : DiscreteIntegrator  ExternalReset=rising  SampleTime=0.1  LimitOutput=on  LowerSaturationLimit=0  ICPrevOutput=DiscIntNeverNeededParam  ICPrevScaledInput=DiscIntNeverNeededParam
  DownshiftInhibitTime : Lookup_n-D  NumberOfTableDimensions=1  BreakpointsForDimension1=[1:1:10]  BreakpointsForDimension2=[1:3]  BeginIndexSearchUsingPreviousIndexResult=on  Table=1.*ones(1,10)  ExtrapMethod=Clip  UseLastTableValue=on  RndMeth=Simplest  InputSameDT=on
  Logical Operator : Logic  AllPortsSameDT=off  OutDataTypeStr=boolean
  Logical Operator1 : Logic  AllPortsSameDT=off  OutDataTypeStr=boolean
  Logical Operator2 : Logic  AllPortsSameDT=off  OutDataTypeStr=boolean
  Relational Operator : RelationalOperator  Operator=<  OutDataTypeStr=boolean  RndMeth=Nearest
  Relational Operator1 : RelationalOperator  OutDataTypeStr=boolean  RndMeth=Nearest
  Relational Operator2 : RelationalOperator  Operator=>  OutDataTypeStr=boolean  RndMeth=Nearest
  Relational Operator3 : RelationalOperator  Operator=>  OutDataTypeStr=boolean  RndMeth=Nearest
  Saturation : Saturate  UpperLimit=6  LowerLimit=1
  Sum1 : Sum  Inputs=++-
  Switch : Switch  Criteria=u2 ~= 0
  Switch1 : Switch  Criteria=u2 ~= 0
  To Workspace1 : ToWorkspace  VariableName=Down  SaveFormat=Timeseries  SampleTime=-1
  To Workspace2 : ToWorkspace  VariableName=UP  SaveFormat=Timeseries  SampleTime=-1
  To Workspace3 : ToWorkspace  VariableName=UpshiftReq  SaveFormat=Timeseries  SampleTime=-1
  To Workspace4 : ToWorkspace  VariableName=DownshiftReq  SaveFormat=Timeseries  SampleTime=-1
  To Workspace5 : ToWorkspace  VariableName=veh_speed  SaveFormat=Timeseries  SampleTime=-1
  To Workspace6 : ToWorkspace  VariableName=up_speed  SaveFormat=Timeseries  SampleTime=-1
  To Workspace7 : ToWorkspace  VariableName=down_speed  SaveFormat=Timeseries  SampleTime=-1
  Unit Delay : UnitDelay  SampleTime=-1
  Unit Delay1 : UnitDelay  SampleTime=-1
  UpshiftInhibitTime : Lookup_n-D  NumberOfTableDimensions=1  BreakpointsForDimension1=[1:1:10]  BreakpointsForDimension2=[1:3]  BeginIndexSearchUsingPreviousIndexResult=on  Table=1.*ones(1,10)  ExtrapMethod=Clip  UseLastTableValue=on  RndMeth=Simplest  InputSameDT=on
  ScheduledRange : Outport
  wires:
  VehicleSpeed_mps/1 -> To Workspace5/1, Relational Operator1/1, Relational Operator/1
  Constant3/1 -> Switch1/3, Switch/3
  Constant2/1 -> Switch1/1
  Constant1/1 -> Switch/1
  Saturation/1 -> ScheduledRange/1  "ScheduledRange"
  UpShiftSpeed/1 -> To Workspace6/1, Relational Operator1/2
  DownShiftSpeed/1 -> To Workspace7/1, Relational Operator/2
  PreviousScheduledRange/1 -> [PrevSchedRng]
  [PrevSchedRng] -> DownshiftInhibitTime/1, UpshiftInhibitTime/1
  Switch/1 -> [UpshiftReq], To Workspace3/1, Sum1/2
  [PrevSchedRng] -> Sum1/1
  Switch1/1 -> [DownshiftReq], To Workspace4/1, Sum1/3
  Sum1/1 -> Saturation/1
  Relational Operator1/1 -> Logical Operator/1
  [AllowUpshift] -> Logical Operator/2
  Relational Operator/1 -> Logical Operator1/1
  [AllowDownshift] -> Logical Operator1/2
  Constant5/1 -> Discrete-Time Integrator/1
  Discrete-Time Integrator/1 -> To Workspace2/1, Relational Operator2/1
  [DownshiftReq] -> Unit Delay/1
  UpshiftInhibitTime/1 -> [UpshiftDelay]
  Relational Operator2/1 -> Logical Operator2/1
  Constant4/1 -> Discrete-Time Integrator1/1
  Discrete-Time Integrator1/1 -> To Workspace1/1, Relational Operator3/1
  [UpshiftReq] -> Unit Delay1/1
  Relational Operator3/1 -> Logical Operator2/2
  DownshiftInhibitTime/1 -> [DownshiftDelay]
  Logical Operator/1 -> Switch/2
  Logical Operator1/1 -> Switch1/2
  [UpshiftDelay] -> Relational Operator2/2
  [DownshiftDelay] -> Relational Operator3/2
  Unit Delay/1 -> Discrete-Time Integrator/2
  Unit Delay1/1 -> Discrete-Time Integrator1/2
  Logical Operator2/1 -> [AllowDownshift], [AllowUpshift]

== matlab function sim/Powertrain Control/TC_Lock_logic ==
  data: VEH_v input; y output; gear input
function y = lock(VEH_v,gear)
%#codegen
if gear >1
    lock =1;
else
    lock =0;
end
y = lock;
